simulink model "B1_pitch_controller_f16"  (R2021b)
settings: Solver=FixedStepAuto  StartTime=0.0  StopTime=10.0  FixedStep=0.0001  RelTol=1e-3
values from neighbouring files (symbols this model uses):
  A_nu = Cmq    [A1_setup_script.m]
  B_nu = Cme    [A1_setup_script.m]
  Cma = A_sp(2,1)    [A1_setup_script.m]
  Cme = B_sp(2,1)    [A1_setup_script.m]
  Cmq = A_sp(2,2)    [A1_setup_script.m]
  CZa = A_sp(1,1)    [A1_setup_script.m]
  filter_cutoff = 2*pi*100    (= 628.318530718)    [A1_setup_script.m]
  filters_on = 1    [A1_setup_script.m]
  Ke = 1/te    (= 10)    [A1_setup_script.m]
  sample_time = 0.002    [A1_setup_script.m]
undefined symbols (not defined in the file or in its folder): DiscIntNeverNeededParam
libraries: cstblocks x2, simulink x1
settings Model: Creator=pieca  LastModifiedBy=pcampolucci

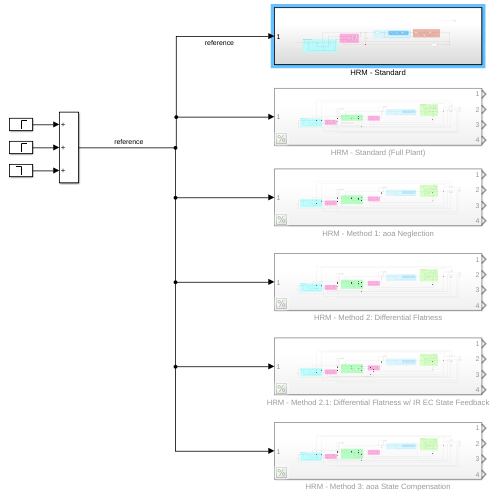
[thumbnail: Simulink's stored preview of the top-level diagram]
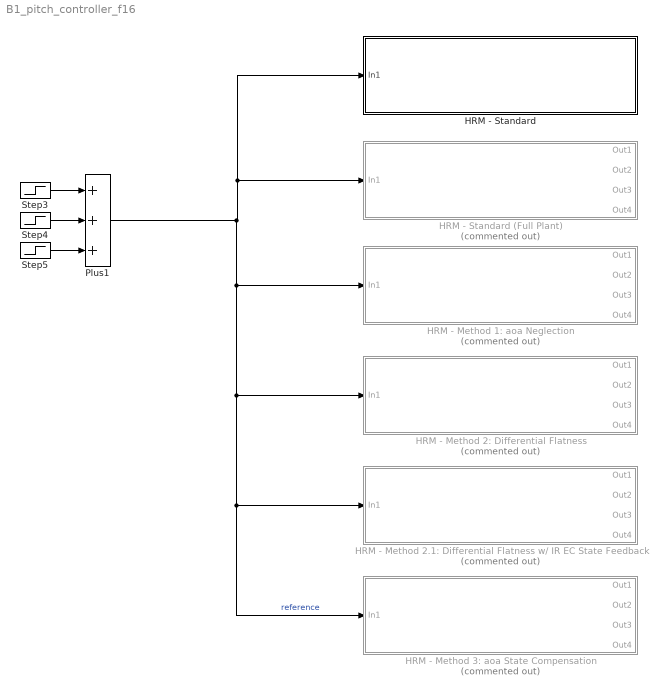
== system B1_pitch_controller_f16 ==
  HRM - Method 1: aoa Neglection : Subsystem  Commented=on
  HRM - Method 2.1: Differential Flatness w/ IR EC State Feedback : Subsystem  Commented=on
  HRM - Method 2: Differential Flatness : Subsystem  Commented=on
  HRM - Method 3: aoa State Compensation : Subsystem  Commented=on
  HRM - Standard : Subsystem
  HRM - Standard (Full Plant) : Subsystem  Commented=on
  Plus1 : Sum  Inputs=+++
  Step3 : Step  After=2  SampleTime=0
  Step4 : Step  Time=4  After=5  SampleTime=0
  Step5 : Step  Time=5.2  After=-3  SampleTime=0
  wires:
  Plus1/1 -> HRM - Method 3: aoa State Compensation/1(In1), HRM - Method 2.1: Differential Flatness w/ IR EC State Feedback/1(In1), HRM - Method 2: Differential Flatness/1(In1), HRM - Method 1: aoa Neglection/1(In1), HRM - Standard/1(In1), HRM - Standard (Full Plant)/1(In1)  "reference"
  Step4/1 -> Plus1/2
  Step5/1 -> Plus1/3
  Step3/1 -> Plus1/1

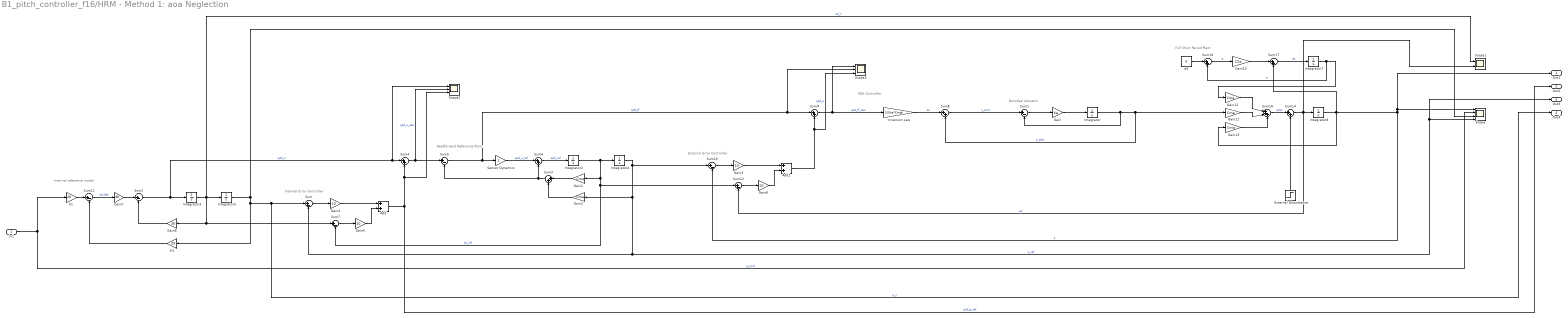
== system B1_pitch_controller_f16/HRM - Method 1: aoa Neglection ==
  note: INDI Controller
  note: Internal Error Controller
  note: NonIdeal Actuator
  note: Internal reference model
  note: External Error Controller
  note: Feedforward Reference Plant
  note: Full Short Period Plant
  In1 : Inport
  -K1 : Gain  Gain=20
  Add : Sum
  Add1 : Sum
  External Disturbance : Step  Time=7  After=10  SampleTime=0
  Gain : Gain  Gain=Ke
  Gain1 : Gain  Gain=Cmq
  Gain10 : Gain  Gain=CZa
  Gain11 : Gain  Gain=Cme
  Gain12 : Gain  Gain=Cma
  Gain13 : Gain  Gain=Cmq
  Gain2 : Gain  Gain=Cma
  Gain{3..6} (4 alike) : Gain  Gain=10
  Gain7 : Gain  Gain=30
  Gain8 : Gain  Gain=30
  Integrator{,2..5,7..8} (7 alike) : Integrator
  Inversion Law : Gain  Gain=1/(Ke*Cme)
  K1 : Gain  Gain=20
  Scope : Scope  NumInputPorts=4
  Scope1 : Scope  NumInputPorts=2
  Scope2 : Scope  NumInputPorts=3
  Scope3 : Scope  NumInputPorts=3
  Sensor Dynamics : Gain
  Sum{,1..2,5,7,10..12} (8 alike) : Sum  Inputs=|+-
  Sum{3..4,6,8..9,14,16..17} (8 alike) : Sum  Inputs=|++
  Sum18 : Sum  Inputs=|+++
  a0 : Constant  Value=0
  Out1 : Outport
  Out2 : Outport  Port=2
  Out3 : Outport  Port=3
  Out4 : Outport  Port=4
  wires:
  Sum3/1 -> Sum5/2, Sum6/2
  Sum8/1 -> Sum1/1  "u_cmd"
  Integrator2/1 -> Integrator4/1, Gain1/1, Sum12/1, Sum7/2  "qd_ref"
  Add/1 -> Scope2/3, Sum4/2, Out2/1  "qdd_e_ref"
  Gain4/1 -> Add/1
  Gain5/1 -> Add/2
  Sensor Dynamics/1 -> Sum6/1  "qdd_u_ref"
  Gain1/1 -> Sum3/1
  Sum6/1 -> Integrator2/1  "qdd_ref"
  Integrator5/1 -> -K1/1, Out4/1, Sum/1, Scope/3  "q_ir"
  K1/1 -> Sum11/1
  Sum4/1 -> Scope2/2, Sum5/1  "qdd_ir_des"
  Integrator3/1 -> Scope1/1, Integrator5/1, Sum7/1, Gain8/1  "qd_ir"
  Gain8/1 -> Sum2/2
  Gain7/1 -> Sum2/1
  Sum1/1 -> Gain/1
  In1/1 -> Scope/2, K1/1  "q_cmd"
  Sum2/1 -> Scope2/1, Sum4/1, Integrator3/1  "qdd_ir"
  Sum12/1 -> Gain6/1
  Sum5/1 -> Scope3/2, Sum9/1, Sensor Dynamics/1  "qdd_ff"
  Add1/1 -> Sum9/2, Scope3/3  "qdd_e"
  Inversion Law/1 -> Sum8/1  "du"
  Gain6/1 -> Add1/2
  Integrator4/1 -> Out3/1, Scope/4, Sum/2, Gain2/1, Sum10/1  "q_ref"
  Sum7/1 -> Gain5/1
  Sum11/1 -> Gain7/1  "qd_des"
  Sum10/1 -> Gain3/1
  Sum9/1 -> Scope3/1, Inversion Law/1  "qdd_ff_des"
  Gain/1 -> Integrator/1
  Gain3/1 -> Add1/1
  Sum/1 -> Gain4/1
  -K1/1 -> Sum11/2
  Sum17/1 -> Integrator7/1  "da"
  Integrator/1 -> Gain11/1, Sum8/2, Sum1/2  "e_elev"
  Sum16/1 -> Gain10/1  "a"
  Integrator8/1 -> Sum17/2, Sum10/2, Scope/1, Out1/1, Gain13/1  "q"
  Sum18/1 -> Sum14/1  "qdot"
  Gain13/1 -> Sum18/3
  Gain12/1 -> Sum18/1
  Gain11/1 -> Sum18/2
  a0/1 -> Sum16/1
  Gain10/1 -> Sum17/1
  Integrator7/1 -> Gain12/1, Sum16/2  "a"
  Sum14/1 -> Sum12/2, Integrator8/1, Scope1/2  "qd"
  External Disturbance/1 -> Sum14/2
  Gain2/1 -> Sum3/2

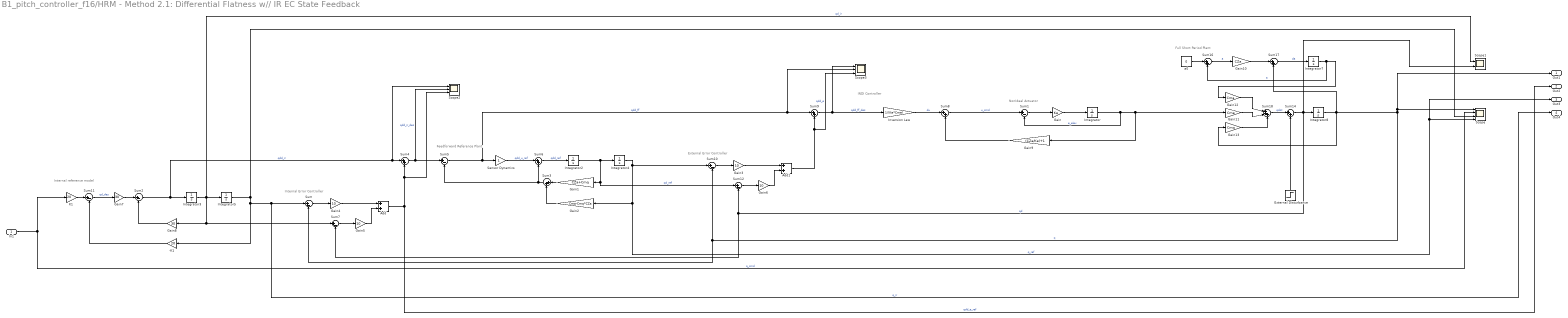
== system B1_pitch_controller_f16/HRM - Method 2.1: Differential Flatness w// IR EC State Feedback ==
  note: INDI Controller
  note: Internal Error Controller
  note: NonIdeal Actuator
  note: Internal reference model
  note: External Error Controller
  note: Feedforward Reference Plant
  note: Full Short Period Plant
  In1 : Inport
  -K1 : Gain  Gain=20
  Add : Sum
  Add1 : Sum
  External Disturbance : Step  Time=7  After=10  SampleTime=0
  Gain : Gain  Gain=Ke
  Gain1 : Gain  Gain=CZa+Cmq
  Gain10 : Gain  Gain=CZa
  Gain11 : Gain  Gain=Cme
  Gain12 : Gain  Gain=Cma
  Gain13 : Gain  Gain=Cmq
  Gain2 : Gain  Gain=Cma-Cmq*CZa
  Gain{3..6} (4 alike) : Gain  Gain=10
  Gain7 : Gain  Gain=30
  Gain8 : Gain  Gain=30
  Gain9 : Gain  Gain=(CZa/Ke)+1
  Integrator{,2..5,7..8} (7 alike) : Integrator
  Inversion Law : Gain  Gain=1/(Ke*Cme)
  K1 : Gain  Gain=20
  Scope : Scope  NumInputPorts=4
  Scope1 : Scope  NumInputPorts=2
  Scope2 : Scope  NumInputPorts=3
  Scope3 : Scope  NumInputPorts=3
  Sensor Dynamics : Gain
  Sum{,1..2,5,7,10..12} (8 alike) : Sum  Inputs=|+-
  Sum{3..4,6,8..9,14,16..17} (8 alike) : Sum  Inputs=|++
  Sum18 : Sum  Inputs=|+++
  a0 : Constant  Value=0
  Out1 : Outport
  Out2 : Outport  Port=2
  Out3 : Outport  Port=3
  Out4 : Outport  Port=4
  wires:
  Sum3/1 -> Sum5/2, Sum6/2
  Sum8/1 -> Sum1/1  "u_cmd"
  Integrator2/1 -> Integrator4/1, Sum12/1, Gain1/1  "qd_ref"
  Add/1 -> Scope2/3, Sum4/2, Out2/1  "qdd_e_ref"
  Gain4/1 -> Add/1
  Gain5/1 -> Add/2
  Sensor Dynamics/1 -> Sum6/1  "qdd_u_ref"
  Sum6/1 -> Integrator2/1  "qdd_ref"
  Integrator5/1 -> -K1/1, Out4/1, Sum/1, Scope/3  "q_ir"
  K1/1 -> Sum11/1
  Sum4/1 -> Scope2/2, Sum5/1  "qdd_ir_des"
  Integrator3/1 -> Scope1/1, Integrator5/1, Sum7/1, Gain8/1  "qd_ir"
  Gain8/1 -> Sum2/2
  Gain7/1 -> Sum2/1
  Sum1/1 -> Gain/1
  In1/1 -> Scope/2, K1/1  "q_cmd"
  Sum2/1 -> Scope2/1, Sum4/1, Integrator3/1  "qdd_ir"
  Sum12/1 -> Gain6/1
  Sum5/1 -> Scope3/2, Sum9/1, Sensor Dynamics/1  "qdd_ff"
  Add1/1 -> Sum9/2, Scope3/3  "qdd_e"
  Inversion Law/1 -> Sum8/1  "du"
  Gain6/1 -> Add1/2
  Integrator4/1 -> Gain2/1, Out3/1, Scope/4, Sum10/1  "q_ref"
  Sum7/1 -> Gain5/1
  Sum11/1 -> Gain7/1  "qd_des"
  Sum10/1 -> Gain3/1
  Sum9/1 -> Scope3/1, Inversion Law/1  "qdd_ff_des"
  Gain/1 -> Integrator/1
  Gain3/1 -> Add1/1
  Sum/1 -> Gain4/1
  -K1/1 -> Sum11/2
  Sum17/1 -> Integrator7/1  "da"
  Integrator/1 -> Gain11/1, Gain9/1, Sum1/2  "e_elev"
  Sum16/1 -> Gain10/1  "a"
  Integrator8/1 -> Sum17/2, Sum/2, Sum10/2, Scope/1, Out1/1, Gain13/1  "q"
  Sum18/1 -> Sum14/1  "qdot"
  Gain13/1 -> Sum18/3
  Gain12/1 -> Sum18/1
  Gain11/1 -> Sum18/2
  a0/1 -> Sum16/1
  Gain10/1 -> Sum17/1
  Integrator7/1 -> Gain12/1, Sum16/2  "a"
  Sum14/1 -> Sum7/2, Sum12/2, Integrator8/1, Scope1/2  "qd"
  External Disturbance/1 -> Sum14/2
  Gain1/1 -> Sum3/1
  Gain2/1 -> Sum3/2
  Gain9/1 -> Sum8/2

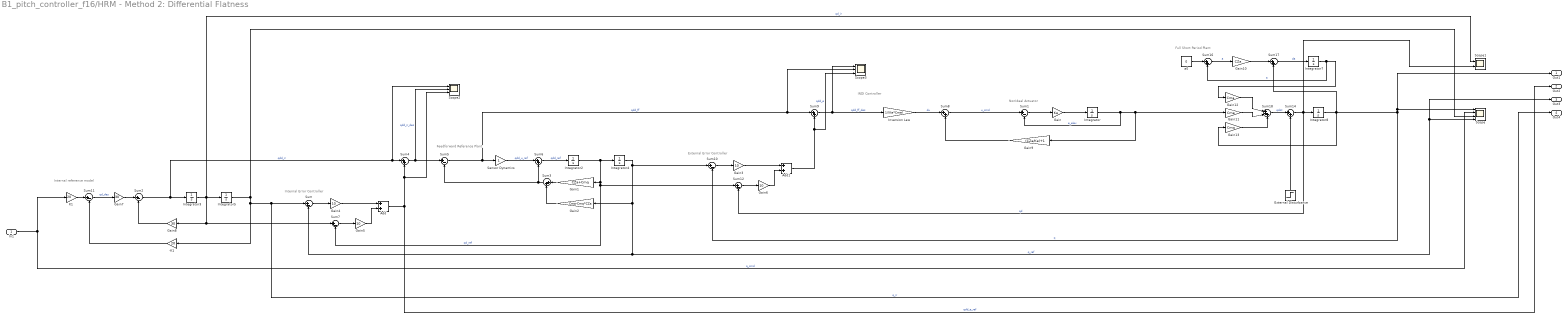
== system B1_pitch_controller_f16/HRM - Method 2: Differential Flatness ==
  note: INDI Controller
  note: Internal Error Controller
  note: NonIdeal Actuator
  note: Internal reference model
  note: External Error Controller
  note: Feedforward Reference Plant
  note: Full Short Period Plant
  In1 : Inport
  -K1 : Gain  Gain=20
  Add : Sum
  Add1 : Sum
  External Disturbance : Step  Time=7  After=10  SampleTime=0
  Gain : Gain  Gain=Ke
  Gain1 : Gain  Gain=CZa+Cmq
  Gain10 : Gain  Gain=CZa
  Gain11 : Gain  Gain=Cme
  Gain12 : Gain  Gain=Cma
  Gain13 : Gain  Gain=Cmq
  Gain2 : Gain  Gain=Cma-Cmq*CZa
  Gain{3..6} (4 alike) : Gain  Gain=10
  Gain7 : Gain  Gain=30
  Gain8 : Gain  Gain=30
  Gain9 : Gain  Gain=(CZa/Ke)+1
  Integrator{,2..5,7..8} (7 alike) : Integrator
  Inversion Law : Gain  Gain=1/(Ke*Cme)
  K1 : Gain  Gain=20
  Scope : Scope  NumInputPorts=4
  Scope1 : Scope  NumInputPorts=2
  Scope2 : Scope  NumInputPorts=3
  Scope3 : Scope  NumInputPorts=3
  Sensor Dynamics : Gain
  Sum{,1..2,5,7,10..12} (8 alike) : Sum  Inputs=|+-
  Sum{3..4,6,8..9,14,16..17} (8 alike) : Sum  Inputs=|++
  Sum18 : Sum  Inputs=|+++
  a0 : Constant  Value=0
  Out1 : Outport
  Out2 : Outport  Port=2
  Out3 : Outport  Port=3
  Out4 : Outport  Port=4
  wires:
  Sum3/1 -> Sum5/2, Sum6/2
  Sum8/1 -> Sum1/1  "u_cmd"
  Integrator2/1 -> Integrator4/1, Sum7/2, Sum12/1, Gain1/1  "qd_ref"
  Add/1 -> Scope2/3, Sum4/2, Out2/1  "qdd_e_ref"
  Gain4/1 -> Add/1
  Gain5/1 -> Add/2
  Sensor Dynamics/1 -> Sum6/1  "qdd_u_ref"
  Sum6/1 -> Integrator2/1  "qdd_ref"
  Integrator5/1 -> -K1/1, Out4/1, Sum/1, Scope/3  "q_ir"
  K1/1 -> Sum11/1
  Sum4/1 -> Scope2/2, Sum5/1  "qdd_ir_des"
  Integrator3/1 -> Scope1/1, Integrator5/1, Sum7/1, Gain8/1  "qd_ir"
  Gain8/1 -> Sum2/2
  Gain7/1 -> Sum2/1
  Sum1/1 -> Gain/1
  In1/1 -> Scope/2, K1/1  "q_cmd"
  Sum2/1 -> Scope2/1, Sum4/1, Integrator3/1  "qdd_ir"
  Sum12/1 -> Gain6/1
  Sum5/1 -> Scope3/2, Sum9/1, Sensor Dynamics/1  "qdd_ff"
  Add1/1 -> Sum9/2, Scope3/3  "qdd_e"
  Inversion Law/1 -> Sum8/1  "du"
  Gain6/1 -> Add1/2
  Integrator4/1 -> Gain2/1, Out3/1, Scope/4, Sum/2, Sum10/1  "q_ref"
  Sum7/1 -> Gain5/1
  Sum11/1 -> Gain7/1  "qd_des"
  Sum10/1 -> Gain3/1
  Sum9/1 -> Scope3/1, Inversion Law/1  "qdd_ff_des"
  Gain/1 -> Integrator/1
  Gain3/1 -> Add1/1
  Sum/1 -> Gain4/1
  -K1/1 -> Sum11/2
  Sum17/1 -> Integrator7/1  "da"
  Integrator/1 -> Gain11/1, Gain9/1, Sum1/2  "e_elev"
  Sum16/1 -> Gain10/1  "a"
  Integrator8/1 -> Sum17/2, Sum10/2, Scope/1, Out1/1, Gain13/1  "q"
  Sum18/1 -> Sum14/1  "qdot"
  Gain13/1 -> Sum18/3
  Gain12/1 -> Sum18/1
  Gain11/1 -> Sum18/2
  a0/1 -> Sum16/1
  Gain10/1 -> Sum17/1
  Integrator7/1 -> Gain12/1, Sum16/2  "a"
  Sum14/1 -> Sum12/2, Integrator8/1, Scope1/2  "qd"
  External Disturbance/1 -> Sum14/2
  Gain1/1 -> Sum3/1
  Gain2/1 -> Sum3/2
  Gain9/1 -> Sum8/2

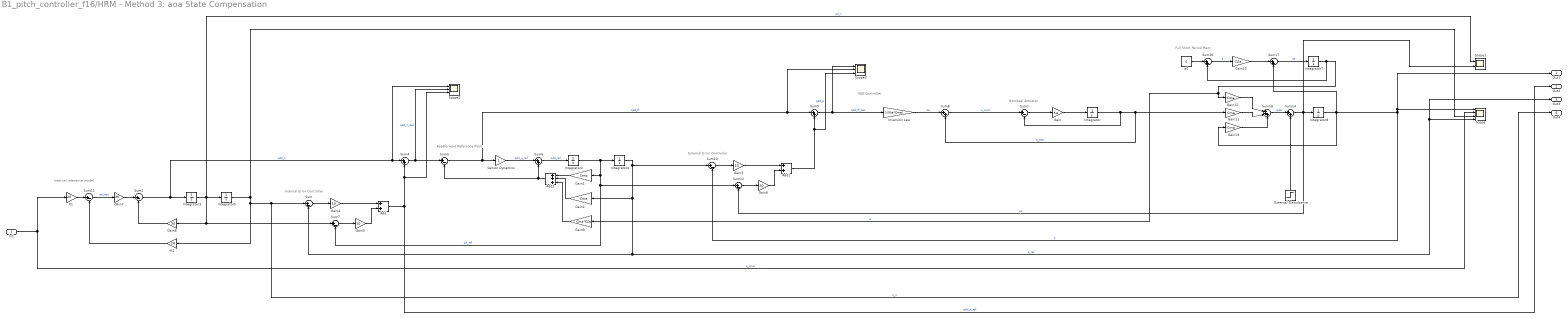
== system B1_pitch_controller_f16/HRM - Method 3: aoa State Compensation ==
  note: INDI Controller
  note: Internal Error Controller
  note: NonIdeal Actuator
  note: Internal reference model
  note: External Error Controller
  note: Feedforward Reference Plant
  note: Full Short Period Plant
  In1 : Inport
  -K1 : Gain  Gain=20
  Add : Sum
  Add1 : Sum
  Add2 : Sum  Inputs=+++
  External Disturbance : Step  Time=7  After=10  SampleTime=0
  Gain : Gain  Gain=Ke
  Gain1 : Gain  Gain=Cmq
  Gain10 : Gain  Gain=CZa
  Gain11 : Gain  Gain=Cme
  Gain12 : Gain  Gain=Cma
  Gain13 : Gain  Gain=Cmq
  Gain2 : Gain  Gain=Cma
  Gain{3..6} (4 alike) : Gain  Gain=10
  Gain7 : Gain  Gain=30
  Gain8 : Gain  Gain=30
  Gain9 : Gain  Gain=Cma*CZa
  Integrator{,2..5,7..8} (7 alike) : Integrator
  Inversion Law : Gain  Gain=1/(Ke*Cme)
  K1 : Gain  Gain=20
  Scope : Scope  NumInputPorts=4
  Scope1 : Scope  NumInputPorts=2
  Scope2 : Scope  NumInputPorts=3
  Scope3 : Scope  NumInputPorts=3
  Sensor Dynamics : Gain
  Sum{,1..2,5,7,10..12} (8 alike) : Sum  Inputs=|+-
  Sum{4,6,8..9,14,16..17} (7 alike) : Sum  Inputs=|++
  Sum18 : Sum  Inputs=|+++
  a0 : Constant  Value=0
  Out1 : Outport
  Out2 : Outport  Port=2
  Out3 : Outport  Port=3
  Out4 : Outport  Port=4
  wires:
  Add2/1 -> Sum5/2, Sum6/2
  Sum8/1 -> Sum1/1  "u_cmd"
  Integrator2/1 -> Integrator4/1, Sum12/1, Sum7/2, Gain1/1  "qd_ref"
  Add/1 -> Scope2/3, Sum4/2, Out2/1  "qdd_e_ref"
  Gain4/1 -> Add/1
  Gain5/1 -> Add/2
  Sensor Dynamics/1 -> Sum6/1  "qdd_u_ref"
  Sum6/1 -> Integrator2/1  "qdd_ref"
  Integrator5/1 -> -K1/1, Out4/1, Sum/1, Scope/3  "q_ir"
  K1/1 -> Sum11/1
  Sum4/1 -> Scope2/2, Sum5/1  "qdd_ir_des"
  Integrator3/1 -> Scope1/1, Integrator5/1, Sum7/1, Gain8/1  "qd_ir"
  Gain8/1 -> Sum2/2
  Gain7/1 -> Sum2/1
  Sum1/1 -> Gain/1
  In1/1 -> Scope/2, K1/1  "q_cmd"
  Sum2/1 -> Scope2/1, Sum4/1, Integrator3/1  "qdd_ir"
  Sum12/1 -> Gain6/1
  Sum5/1 -> Scope3/2, Sum9/1, Sensor Dynamics/1  "qdd_ff"
  Add1/1 -> Sum9/2, Scope3/3  "qdd_e"
  Inversion Law/1 -> Sum8/1  "du"
  Gain6/1 -> Add1/2
  Integrator4/1 -> Out3/1, Scope/4, Sum/2, Gain2/1, Sum10/1  "q_ref"
  Sum7/1 -> Gain5/1
  Sum11/1 -> Gain7/1  "qd_des"
  Sum10/1 -> Gain3/1
  Sum9/1 -> Scope3/1, Inversion Law/1  "qdd_ff_des"
  Gain/1 -> Integrator/1
  Gain3/1 -> Add1/1
  Sum/1 -> Gain4/1
  -K1/1 -> Sum11/2
  Sum17/1 -> Integrator7/1  "da"
  Integrator/1 -> Gain11/1, Sum8/2, Sum1/2  "e_elev"
  Sum16/1 -> Gain10/1  "a"
  Integrator8/1 -> Sum17/2, Sum10/2, Scope/1, Out1/1, Gain13/1  "q"
  Sum18/1 -> Sum14/1  "qdot"
  Gain13/1 -> Sum18/3
  Gain12/1 -> Sum18/1
  Gain11/1 -> Sum18/2
  a0/1 -> Sum16/1
  Gain10/1 -> Sum17/1
  Integrator7/1 -> Gain9/1, Gain12/1, Sum16/2  "a"
  Sum14/1 -> Sum12/2, Integrator8/1, Scope1/2  "qd"
  External Disturbance/1 -> Sum14/2
  Gain1/1 -> Add2/1
  Gain2/1 -> Add2/2
  Gain9/1 -> Add2/3

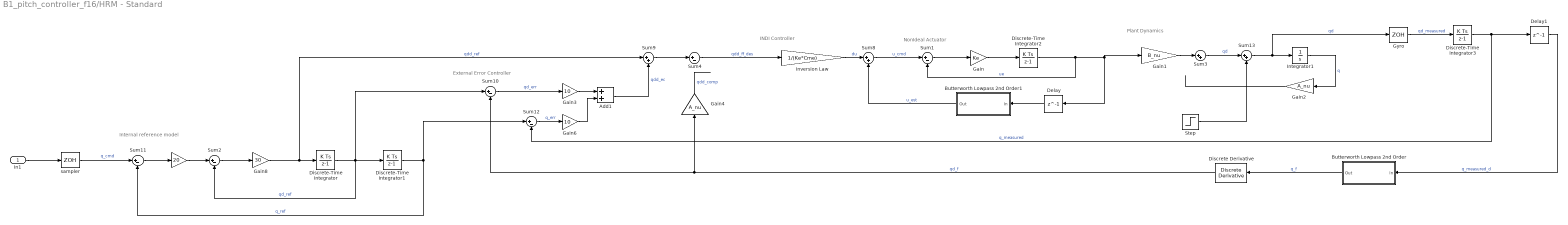
== system B1_pitch_controller_f16/HRM - Standard ==
  note: INDI Controller
  note: NonIdeal Actuator
  note: Internal reference model
  note: External Error Controller
  note: Plant Dynamics
  In1 : Inport
  "  " : Gain  Gain=20
  Add1 : Sum
  Butterworth Lowpass 2nd Order : Subsystem
  Butterworth Lowpass 2nd Order1 : Subsystem
  Delay : Delay  DelayLength=1  SampleTime=sample_time
  Delay1 : Delay  DelayLength=1  SampleTime=sample_time
  Discrete Derivative : simulink/Discrete/Discrete Derivative  gainval=1.0  ICPrevScaledInput=0.0  OutMin=[]  OutMax=[]  OutDataType=fixdt(1, 16)  OutScaling=2^-10  DoSatur=off
  Discrete-Time Integrator{,1..3} (4 alike) : DiscreteIntegrator  SampleTime=-1  ICPrevOutput=DiscIntNeverNeededParam  ICPrevScaledInput=DiscIntNeverNeededParam
  Gain : Gain  Gain=Ke
  Gain1 : Gain  Gain=B_nu
  Gain2 : Gain  Gain=A_nu
  Gain3 : Gain  Gain=10
  Gain4 : Gain  Gain=A_nu
  Gain6 : Gain  Gain=10
  Gain8 : Gain  Gain=30
  Gyro : ZeroOrderHold  SampleTime=sample_time
  Integrator1 : Integrator
  Inversion Law : Gain  Gain=1/(Ke*Cme)
  Step : Step  Time=6  After=10  SampleTime=0
  Sum{1..2,4,10..12} (6 alike) : Sum  Inputs=|+-
  Sum{3,8..9,13} (4 alike) : Sum  Inputs=|++
  sampler : ZeroOrderHold  SampleTime=sample_time
  wires:
  Sum13/1 -> Gyro/1, Integrator1/1  "qd"
  Sum8/1 -> Sum1/1  "u_cmd"
  Integrator1/1 -> Gain2/1  "q"
  Gain1/1 -> Sum3/1
  Discrete-Time Integrator1/1 -> Sum11/2, Sum12/1  "q_ref"
  Discrete-Time Integrator/1 -> Sum2/2, Discrete-Time Integrator1/1, Sum10/1  "qd_ref"
  "  "/1 -> Sum2/1
  Sum1/1 -> Gain/1
  sampler/1 -> Sum11/1  "q_cmd"
  Sum2/1 -> Gain8/1
  Sum12/1 -> Gain6/1  "q_err"
  Add1/1 -> Sum9/2  "qdd_ec"
  Inversion Law/1 -> Sum8/1  "du"
  Sum3/1 -> Sum13/1  "qd"
  Discrete-Time Integrator2/1 -> Gain1/1, Delay/1, Sum1/2  "ue"
  Gain6/1 -> Add1/2
  Gain2/1 -> ?
  Sum11/1 -> "  "/1
  Sum10/1 -> Gain3/1  "qd_err"
  Sum4/1 -> Inversion Law/1  "qdd_ff_des"
  Gain/1 -> Discrete-Time Integrator2/1
  Gain3/1 -> Add1/1
  Sum9/1 -> Sum4/1
  Gain4/1 -> ?  "qdd_comp"
  In1/1 -> sampler/1
  Butterworth Lowpass 2nd Order1/1(Out) -> Sum8/2  "u_est"
  Delay/1 -> Butterworth Lowpass 2nd Order1/1(In)
  Gyro/1 -> Discrete-Time Integrator3/1  "qd_measured"
  Delay1/1 -> Butterworth Lowpass 2nd Order/1(In)  "q_measured_d"
  Butterworth Lowpass 2nd Order/1(Out) -> Discrete Derivative/1  "q_f"
  Discrete Derivative/1 -> Sum10/2, Gain4/1  "qd_f"
  Discrete-Time Integrator3/1 -> Delay1/1, Sum12/2  "q_measured"
  Gain8/1 -> Sum9/1, Discrete-Time Integrator/1  "qdd_ref"
  Step/1 -> Sum13/2

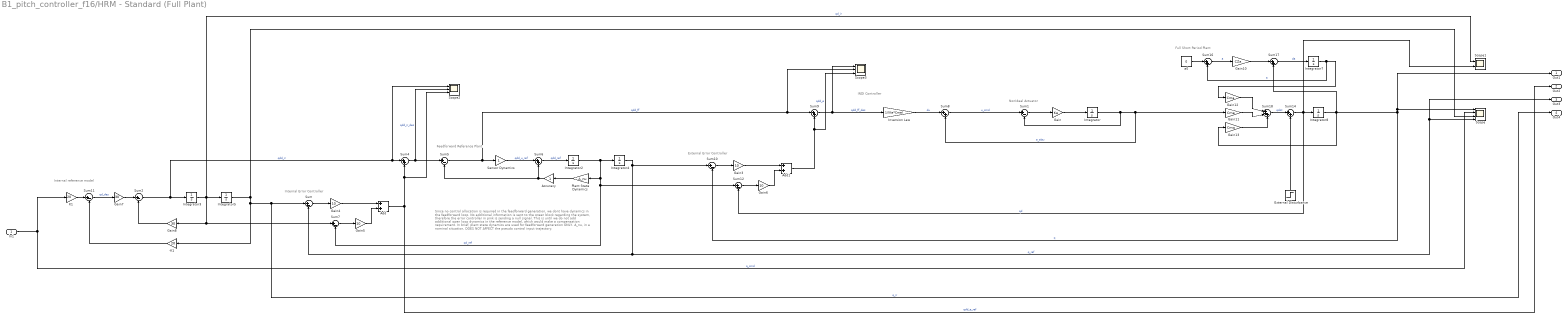
== system B1_pitch_controller_f16/HRM - Standard (Full Plant) ==
  note: Since no control allocation is required in the feedforward generation, we dont have dynamics in the feedforward loop. No additional information is sent to the green block regarding the system, therefore the error controller in pink is sending a null signal. This is until we do not add additional open loop dynamics in the reference model, which would make a compensation requirement. In brief, plant state dynamics are used for feedforward generation ONLY. A_nu, in a nominal situation, DOES NOT AFFECT the pseudo control input trajectory.
  note: INDI Controller
  note: Internal Error Controller
  note: NonIdeal Actuator
  note: Internal reference model
  note: External Error Controller
  note: Feedforward Reference Plant
  note: Full Short Period Plant
  In1 : Inport
  -K1 : Gain  Gain=20
  Accuracy : Gain
  Add : Sum
  Add1 : Sum
  External Disturbance : Step  Time=7  After=10  SampleTime=0
  Gain : Gain  Gain=Ke
  Gain10 : Gain  Gain=CZa
  Gain11 : Gain  Gain=Cme
  Gain12 : Gain  Gain=Cma
  Gain13 : Gain  Gain=Cmq
  Gain{3..6} (4 alike) : Gain  Gain=10
  Gain7 : Gain  Gain=30
  Gain8 : Gain  Gain=30
  Integrator{,2..5,7..8} (7 alike) : Integrator
  Inversion Law : Gain  Gain=1/(Ke*Cme)
  K1 : Gain  Gain=20
  Plant State Dynamics : Gain  Gain=A_nu
  Scope : Scope  NumInputPorts=4
  Scope1 : Scope  NumInputPorts=2
  Scope2 : Scope  NumInputPorts=3
  Scope3 : Scope  NumInputPorts=3
  Sensor Dynamics : Gain
  Sum{,1..2,5,7,10..12} (8 alike) : Sum  Inputs=|+-
  Sum{4,6,8..9,14,16..17} (7 alike) : Sum  Inputs=|++
  Sum18 : Sum  Inputs=|+++
  a0 : Constant  Value=0
  Out1 : Outport
  Out2 : Outport  Port=2
  Out3 : Outport  Port=3
  Out4 : Outport  Port=4
  wires:
  Accuracy/1 -> Sum5/2, Sum6/2
  Sum8/1 -> Sum1/1  "u_cmd"
  Integrator2/1 -> Integrator4/1, Sum12/1, Sum7/2, Plant State Dynamics/1  "qd_ref"
  Add/1 -> Scope2/3, Sum4/2, Out2/1  "qdd_e_ref"
  Gain4/1 -> Add/1
  Gain5/1 -> Add/2
  Sensor Dynamics/1 -> Sum6/1  "qdd_u_ref"
  Plant State Dynamics/1 -> Accuracy/1
  Sum6/1 -> Integrator2/1  "qdd_ref"
  Integrator5/1 -> -K1/1, Out4/1, Sum/1, Scope/3  "q_ir"
  K1/1 -> Sum11/1
  Sum4/1 -> Scope2/2, Sum5/1  "qdd_ir_des"
  Integrator3/1 -> Scope1/1, Integrator5/1, Sum7/1, Gain8/1  "qd_ir"
  Gain8/1 -> Sum2/2
  Gain7/1 -> Sum2/1
  Sum1/1 -> Gain/1
  In1/1 -> Scope/2, K1/1  "q_cmd"
  Sum2/1 -> Scope2/1, Sum4/1, Integrator3/1  "qdd_ir"
  Sum12/1 -> Gain6/1
  Sum5/1 -> Scope3/2, Sum9/1, Sensor Dynamics/1  "qdd_ff"
  Add1/1 -> Sum9/2, Scope3/3  "qdd_e"
  Inversion Law/1 -> Sum8/1  "du"
  Gain6/1 -> Add1/2
  Integrator4/1 -> Out3/1, Scope/4, Sum/2, Sum10/1  "q_ref"
  Sum7/1 -> Gain5/1
  Sum11/1 -> Gain7/1  "qd_des"
  Sum10/1 -> Gain3/1
  Sum9/1 -> Scope3/1, Inversion Law/1  "qdd_ff_des"
  Gain/1 -> Integrator/1
  Gain3/1 -> Add1/1
  Sum/1 -> Gain4/1
  -K1/1 -> Sum11/2
  Sum17/1 -> Integrator7/1  "da"
  Integrator/1 -> Gain11/1, Sum8/2, Sum1/2  "e_elev"
  Sum16/1 -> Gain10/1  "a"
  Integrator8/1 -> Sum17/2, Sum10/2, Scope/1, Out1/1, Gain13/1  "q"
  Sum18/1 -> Sum14/1  "qdot"
  Gain13/1 -> Sum18/3
  Gain12/1 -> Sum18/1
  Gain11/1 -> Sum18/2
  a0/1 -> Sum16/1
  Gain10/1 -> Sum17/1
  Integrator7/1 -> Gain12/1, Sum16/2  "a"
  Sum14/1 -> Sum12/2, Integrator8/1, Scope1/2  "qd"
  External Disturbance/1 -> Sum14/2

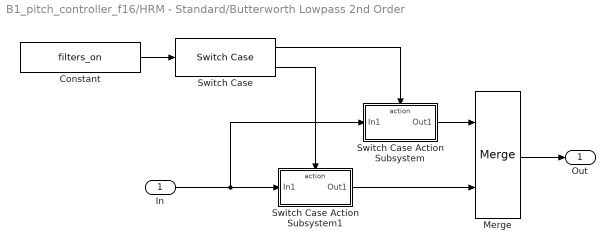
== system B1_pitch_controller_f16/HRM - Standard/Butterworth Lowpass 2nd Order ==
  In : Inport
  Constant : Constant  Value=filters_on  SampleTime=sample_time
  Merge : Merge
  Switch Case : SwitchCase
  Switch Case Action Subsystem : Subsystem  TreatAsAtomicUnit=on
  Switch Case Action Subsystem1 : Subsystem  TreatAsAtomicUnit=on
  Out : Outport
  wires:
  Merge/1 -> Out/1
  Switch Case Action Subsystem/1(Out1) -> Merge/1
  Constant/1 -> Switch Case/1
  Switch Case Action Subsystem1/1(Out1) -> Merge/2
  Switch Case/2 -> Switch Case Action Subsystem1/Action
  In/1 -> Switch Case Action Subsystem/1(In1), Switch Case Action Subsystem1/1(In1)
  Switch Case/1 -> Switch Case Action Subsystem/Action

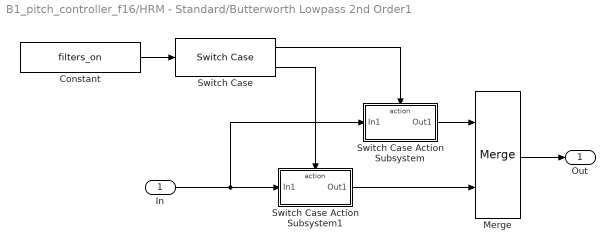
== system B1_pitch_controller_f16/HRM - Standard/Butterworth Lowpass 2nd Order1 ==
  In : Inport
  Constant : Constant  Value=filters_on  SampleTime=sample_time
  Merge : Merge
  Switch Case : SwitchCase
  Switch Case Action Subsystem : Subsystem  TreatAsAtomicUnit=on
  Switch Case Action Subsystem1 : Subsystem  TreatAsAtomicUnit=on
  Out : Outport
  wires:
  Merge/1 -> Out/1
  Switch Case Action Subsystem/1(Out1) -> Merge/1
  Constant/1 -> Switch Case/1
  Switch Case Action Subsystem1/1(Out1) -> Merge/2
  Switch Case/2 -> Switch Case Action Subsystem1/Action
  In/1 -> Switch Case Action Subsystem/1(In1), Switch Case Action Subsystem1/1(In1)
  Switch Case/1 -> Switch Case Action Subsystem/Action

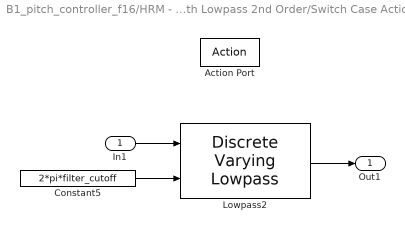
== system B1_pitch_controller_f16/HRM - Standard/Butterworth Lowpass 2nd Order/Switch Case Action Subsystem ==
  In1 : Inport
  Action Port : ActionPort  ActionPortLabel=case [ 1 ]:
  Constant5 : Constant  Value=2*pi*filter_cutoff  SampleTime=sample_time
  Lowpass2 : cstblocks/Linear Parameter Varying/Discrete Varying Lowpass  N=2  w0=0  Ts=sample_time
      settings: SourceProductBaseCode=CT
  Out1 : Outport
  wires:
  Constant5/1 -> Lowpass2/2
  In1/1 -> Lowpass2/1
  Lowpass2/1 -> Out1/1

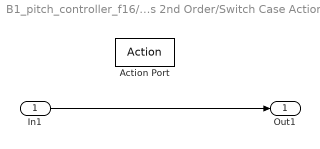
== system B1_pitch_controller_f16/HRM - Standard/Butterworth Lowpass 2nd Order/Switch Case Action Subsystem1 ==
  In1 : Inport
  Action Port : ActionPort  ActionPortLabel=default:
  Out1 : Outport
  wires:
  In1/1 -> Out1/1

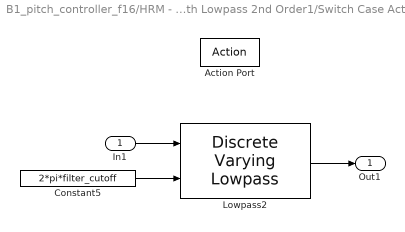
== system B1_pitch_controller_f16/HRM - Standard/Butterworth Lowpass 2nd Order1/Switch Case Action Subsystem ==
  In1 : Inport
  Action Port : ActionPort  ActionPortLabel=case [ 1 ]:
  Constant5 : Constant  Value=2*pi*filter_cutoff  SampleTime=sample_time
  Lowpass2 : cstblocks/Linear Parameter Varying/Discrete Varying Lowpass  N=2  w0=0  Ts=sample_time
      settings: SourceProductBaseCode=CT
  Out1 : Outport
  wires:
  Constant5/1 -> Lowpass2/2
  In1/1 -> Lowpass2/1
  Lowpass2/1 -> Out1/1

== system B1_pitch_controller_f16/HRM - Standard/Butterworth Lowpass 2nd Order1/Switch Case Action Subsystem1 ==
  In1 : Inport
  Action Port : ActionPort  ActionPortLabel=default:
  Out1 : Outport
  wires:
  In1/1 -> Out1/1
